simulink model "b6_formation"  (R2021b)
settings: Solver=FixedStepAuto  StartTime=0.0  StopTime=inf  FixedStep=sampleTime  RelTol=1e-3
PreLoadFcn:
  | % Simulation parameters
  | %load exampleMap
  | 
  | % Lidar parameters
  | sensorOffset = [0,0];
  | scanAngles = -pi/2:pi/6:pi/2;
  | maxRange = 0.3;
InitFcn:
  | sampleTime = 0.05;
  | nMedianSize=3;
  | % Robot parameters
  | wheelRadius = 0.0335;
  | robotRadius = 0.116/2;
  | 
  | %角速度坐标
  | ks=1;
  | 
  | % Lidar parameters
  | sensorOffset = [0,0];
  | scanAngles = -pi:pi/36:pi;
  | maxRange = 0.2;
  | 
  | %车初始位置
  | init_pose_1=[1  1.3  pi/2]';
  | init_pose_2=[0.85 1  pi/2]';
  | init_pose_3=[1.15 1  pi/2]';
  | init_pose_4=[0.7  0.7 pi/2]';
  | init_pose_5=[1  0.7 pi/2]';
  | init_pose_6=[1.3 0.7  pi/2]';
  | 
  | %pp算法性能参数
  | Vd_pp=0.2;
  | Wd_pp=pi;
  | dist_pp=0.2;
  | GoalRadius=0.1;
  | numSector=180;
  | rangeDis=[0.1,maxRange];
  | thresholds=[1/360 1/36];
  | safetyDis=0.2;
  | minimumTurningRadius=0.5*robotRadius;
  | recovery_w=0.05;
undefined symbols (not defined in the file): Angular, DiscIntNeverNeededParam, Linear, Pose, Twist
libraries: robotlib x42, dspstat3 x18, mobileRoboticsLib x7, robotmobilelib x6, robotalgslib x6
(part 2 of 5)

== system b6_formation/Subsystem/Car Pose Listener/Subsystem ==
  poseNew : Inport
  poseMsg : Inport  Port=2
  VW_New : Inport  Port=3
  VW_Msg : Inport  Port=4
  DiffSteer Kinematics : Subsystem
      settings: PortSchema="{\"entries\":[{\"content\":{\"sides\":[{\"content\":{\"connectorIds\":[\"In1\",\"In2\"]},\"type\":\"ConnectorPlacement.EquallySpacedRectSide\",\"uuid\":\"0032ed68-1de4-4b1c-b237-9372fedc8a7a\"},{\"content\":{\"connectorIds\":[\"Out1\",\"Out2\",\"Out3\"],\"side\":\"RIGHT\"},\"type\":\"ConnectorPlacement.EquallySpacedRectSide\",\"uuid\":\"d0c861bd-7497-47fe-b183-36da470ee2c6\"},{\"content\":{\"connectorIds\":[\"In3\",\"In4\"],\"side\":\"TOP\"},\"type\":\"ConnectorPlacement.EquallySpacedRectSide\",\"uuid\":\"5b685229-150b-4cb5-b33d-c61d28c4627e\"}]},\"type\":\"ConnectorPlacement.EquallySpacedConnector\",\"uuid\":\"4513c50b-5820-40cb-bb28-cc7c1b1322fe\"}],\"packageUris\":[\"http://schema.mathworks.com/mf0/Connector/R2020b\"],\"version\":\"1.0\"}"
  Median Filter : dspstat3/Median Filter  WindowLength=nMedianSize  SimulateUsing=Interpreted execution
      settings: SourceProductBaseCode=DS
  Median Filter1 : dspstat3/Median Filter  WindowLength=nMedianSize  SimulateUsing=Interpreted execution
      settings: SourceProductBaseCode=DS
  Median Filter2 : dspstat3/Median Filter  WindowLength=nMedianSize  SimulateUsing=Interpreted execution
      settings: SourceProductBaseCode=DS
  Mux7 : Mux  Inputs=3
  Sum : Sum  Inputs=++|
  Sum1 : Sum  Inputs=++|
  sensor2vCar : MATLAB Function  TreatAsAtomicUnit=on
  sensor2vCar4 : MATLAB Function  TreatAsAtomicUnit=on
  pose : Outport
  wires:
  Median Filter2/1 -> Mux7/3
  Median Filter1/1 -> Mux7/2
  Median Filter/1 -> Mux7/1
  sensor2vCar/4(flag) -> DiffSteer Kinematics/3(reset)
  DiffSteer Kinematics/2(y) -> Sum1/2
  sensor2vCar/3(yaw_init) -> DiffSteer Kinematics/4(yaw0)
  sensor2vCar/2(y_init) -> Sum1/1
  sensor2vCar/1(x_init) -> Sum/1
  DiffSteer Kinematics/1(x) -> Sum/2
  VW_New/1 -> sensor2vCar4/1(VW_New)
  Mux7/1 -> pose/1
  Sum/1 -> Median Filter/1
  DiffSteer Kinematics/3(psi) -> Median Filter2/1
  sensor2vCar4/1(V) -> DiffSteer Kinematics/1(u)
  Sum1/1 -> Median Filter1/1
  sensor2vCar4/2(W) -> DiffSteer Kinematics/2(w)
  poseNew/1 -> sensor2vCar/1(poseNew)
  poseMsg/1 -> sensor2vCar/2(poseMsg)
  VW_Msg/1 -> sensor2vCar4/2(VW_Msg)

== system b6_formation/Subsystem/Car Pose Listener1/Subsystem ==
  poseNew : Inport
  poseMsg : Inport  Port=2
  VW_New : Inport  Port=3
  VW_Msg : Inport  Port=4
  DiffSteer Kinematics : Subsystem
      settings: PortSchema="{\"entries\":[{\"content\":{\"sides\":[{\"content\":{\"connectorIds\":[\"In1\",\"In2\"]},\"type\":\"ConnectorPlacement.EquallySpacedRectSide\",\"uuid\":\"0032ed68-1de4-4b1c-b237-9372fedc8a7a\"},{\"content\":{\"connectorIds\":[\"Out1\",\"Out2\",\"Out3\"],\"side\":\"RIGHT\"},\"type\":\"ConnectorPlacement.EquallySpacedRectSide\",\"uuid\":\"d0c861bd-7497-47fe-b183-36da470ee2c6\"},{\"content\":{\"connectorIds\":[\"In3\",\"In4\"],\"side\":\"TOP\"},\"type\":\"ConnectorPlacement.EquallySpacedRectSide\",\"uuid\":\"5b685229-150b-4cb5-b33d-c61d28c4627e\"}]},\"type\":\"ConnectorPlacement.EquallySpacedConnector\",\"uuid\":\"4513c50b-5820-40cb-bb28-cc7c1b1322fe\"}],\"packageUris\":[\"http://schema.mathworks.com/mf0/Connector/R2020b\"],\"version\":\"1.0\"}"
  Median Filter : dspstat3/Median Filter  WindowLength=nMedianSize  SimulateUsing=Interpreted execution
      settings: SourceProductBaseCode=DS
  Median Filter1 : dspstat3/Median Filter  WindowLength=nMedianSize  SimulateUsing=Interpreted execution
      settings: SourceProductBaseCode=DS
  Median Filter2 : dspstat3/Median Filter  WindowLength=nMedianSize  SimulateUsing=Interpreted execution
      settings: SourceProductBaseCode=DS
  Mux7 : Mux  Inputs=3
  Sum : Sum  Inputs=++|
  Sum1 : Sum  Inputs=++|
  sensor2vCar : MATLAB Function  TreatAsAtomicUnit=on
  sensor2vCar4 : MATLAB Function  TreatAsAtomicUnit=on
  pose : Outport
  wires:
  Median Filter2/1 -> Mux7/3
  Median Filter1/1 -> Mux7/2
  Median Filter/1 -> Mux7/1
  sensor2vCar/4(flag) -> DiffSteer Kinematics/3(reset)
  DiffSteer Kinematics/2(y) -> Sum1/2
  sensor2vCar/3(yaw_init) -> DiffSteer Kinematics/4(yaw0)
  sensor2vCar/2(y_init) -> Sum1/1
  sensor2vCar/1(x_init) -> Sum/1
  DiffSteer Kinematics/1(x) -> Sum/2
  VW_New/1 -> sensor2vCar4/1(VW_New)
  Mux7/1 -> pose/1
  Sum/1 -> Median Filter/1
  DiffSteer Kinematics/3(psi) -> Median Filter2/1
  sensor2vCar4/1(V) -> DiffSteer Kinematics/1(u)
  Sum1/1 -> Median Filter1/1
  sensor2vCar4/2(W) -> DiffSteer Kinematics/2(w)
  poseNew/1 -> sensor2vCar/1(poseNew)
  poseMsg/1 -> sensor2vCar/2(poseMsg)
  VW_Msg/1 -> sensor2vCar4/2(VW_Msg)

== system b6_formation/Subsystem/Car Pose Listener2/Subsystem ==
  poseNew : Inport
  poseMsg : Inport  Port=2
  VW_New : Inport  Port=3
  VW_Msg : Inport  Port=4
  DiffSteer Kinematics : Subsystem
      settings: PortSchema="{\"entries\":[{\"content\":{\"sides\":[{\"content\":{\"connectorIds\":[\"In1\",\"In2\"]},\"type\":\"ConnectorPlacement.EquallySpacedRectSide\",\"uuid\":\"0032ed68-1de4-4b1c-b237-9372fedc8a7a\"},{\"content\":{\"connectorIds\":[\"Out1\",\"Out2\",\"Out3\"],\"side\":\"RIGHT\"},\"type\":\"ConnectorPlacement.EquallySpacedRectSide\",\"uuid\":\"d0c861bd-7497-47fe-b183-36da470ee2c6\"},{\"content\":{\"connectorIds\":[\"In3\",\"In4\"],\"side\":\"TOP\"},\"type\":\"ConnectorPlacement.EquallySpacedRectSide\",\"uuid\":\"5b685229-150b-4cb5-b33d-c61d28c4627e\"}]},\"type\":\"ConnectorPlacement.EquallySpacedConnector\",\"uuid\":\"4513c50b-5820-40cb-bb28-cc7c1b1322fe\"}],\"packageUris\":[\"http://schema.mathworks.com/mf0/Connector/R2020b\"],\"version\":\"1.0\"}"
  Median Filter : dspstat3/Median Filter  WindowLength=nMedianSize  SimulateUsing=Interpreted execution
      settings: SourceProductBaseCode=DS
  Median Filter1 : dspstat3/Median Filter  WindowLength=nMedianSize  SimulateUsing=Interpreted execution
      settings: SourceProductBaseCode=DS
  Median Filter2 : dspstat3/Median Filter  WindowLength=nMedianSize  SimulateUsing=Interpreted execution
      settings: SourceProductBaseCode=DS
  Mux7 : Mux  Inputs=3
  Sum : Sum  Inputs=++|
  Sum1 : Sum  Inputs=++|
  sensor2vCar : MATLAB Function  TreatAsAtomicUnit=on
  sensor2vCar4 : MATLAB Function  TreatAsAtomicUnit=on
  pose : Outport
  wires:
  Median Filter2/1 -> Mux7/3
  Median Filter1/1 -> Mux7/2
  Median Filter/1 -> Mux7/1
  sensor2vCar/4(flag) -> DiffSteer Kinematics/3(reset)
  DiffSteer Kinematics/2(y) -> Sum1/2
  sensor2vCar/3(yaw_init) -> DiffSteer Kinematics/4(yaw0)
  sensor2vCar/2(y_init) -> Sum1/1
  sensor2vCar/1(x_init) -> Sum/1
  DiffSteer Kinematics/1(x) -> Sum/2
  VW_New/1 -> sensor2vCar4/1(VW_New)
  Mux7/1 -> pose/1
  Sum/1 -> Median Filter/1
  DiffSteer Kinematics/3(psi) -> Median Filter2/1
  sensor2vCar4/1(V) -> DiffSteer Kinematics/1(u)
  Sum1/1 -> Median Filter1/1
  sensor2vCar4/2(W) -> DiffSteer Kinematics/2(w)
  poseNew/1 -> sensor2vCar/1(poseNew)
  poseMsg/1 -> sensor2vCar/2(poseMsg)
  VW_Msg/1 -> sensor2vCar4/2(VW_Msg)

== system b6_formation/Subsystem/Car Pose Listener3/Subsystem ==
  poseNew : Inport
  poseMsg : Inport  Port=2
  VW_New : Inport  Port=3
  VW_Msg : Inport  Port=4
  DiffSteer Kinematics : Subsystem
      settings: PortSchema="{\"entries\":[{\"content\":{\"sides\":[{\"content\":{\"connectorIds\":[\"In1\",\"In2\"]},\"type\":\"ConnectorPlacement.EquallySpacedRectSide\",\"uuid\":\"0032ed68-1de4-4b1c-b237-9372fedc8a7a\"},{\"content\":{\"connectorIds\":[\"Out1\",\"Out2\",\"Out3\"],\"side\":\"RIGHT\"},\"type\":\"ConnectorPlacement.EquallySpacedRectSide\",\"uuid\":\"d0c861bd-7497-47fe-b183-36da470ee2c6\"},{\"content\":{\"connectorIds\":[\"In3\",\"In4\"],\"side\":\"TOP\"},\"type\":\"ConnectorPlacement.EquallySpacedRectSide\",\"uuid\":\"5b685229-150b-4cb5-b33d-c61d28c4627e\"}]},\"type\":\"ConnectorPlacement.EquallySpacedConnector\",\"uuid\":\"4513c50b-5820-40cb-bb28-cc7c1b1322fe\"}],\"packageUris\":[\"http://schema.mathworks.com/mf0/Connector/R2020b\"],\"version\":\"1.0\"}"
  Median Filter : dspstat3/Median Filter  WindowLength=nMedianSize  SimulateUsing=Interpreted execution
      settings: SourceProductBaseCode=DS
  Median Filter1 : dspstat3/Median Filter  WindowLength=nMedianSize  SimulateUsing=Interpreted execution
      settings: SourceProductBaseCode=DS
  Median Filter2 : dspstat3/Median Filter  WindowLength=nMedianSize  SimulateUsing=Interpreted execution
      settings: SourceProductBaseCode=DS
  Mux7 : Mux  Inputs=3
  Sum : Sum  Inputs=++|
  Sum1 : Sum  Inputs=++|
  sensor2vCar : MATLAB Function  TreatAsAtomicUnit=on
  sensor2vCar4 : MATLAB Function  TreatAsAtomicUnit=on
  pose : Outport
  wires:
  Median Filter2/1 -> Mux7/3
  Median Filter1/1 -> Mux7/2
  Median Filter/1 -> Mux7/1
  sensor2vCar/4(flag) -> DiffSteer Kinematics/3(reset)
  DiffSteer Kinematics/2(y) -> Sum1/2
  sensor2vCar/3(yaw_init) -> DiffSteer Kinematics/4(yaw0)
  sensor2vCar/2(y_init) -> Sum1/1
  sensor2vCar/1(x_init) -> Sum/1
  DiffSteer Kinematics/1(x) -> Sum/2
  VW_New/1 -> sensor2vCar4/1(VW_New)
  Mux7/1 -> pose/1
  Sum/1 -> Median Filter/1
  DiffSteer Kinematics/3(psi) -> Median Filter2/1
  sensor2vCar4/1(V) -> DiffSteer Kinematics/1(u)
  Sum1/1 -> Median Filter1/1
  sensor2vCar4/2(W) -> DiffSteer Kinematics/2(w)
  poseNew/1 -> sensor2vCar/1(poseNew)
  poseMsg/1 -> sensor2vCar/2(poseMsg)
  VW_Msg/1 -> sensor2vCar4/2(VW_Msg)

== system b6_formation/Subsystem/Car Pose Listener4/Subsystem ==
  poseNew : Inport
  poseMsg : Inport  Port=2
  VW_New : Inport  Port=3
  VW_Msg : Inport  Port=4
  DiffSteer Kinematics : Subsystem
      settings: PortSchema="{\"entries\":[{\"content\":{\"sides\":[{\"content\":{\"connectorIds\":[\"In1\",\"In2\"]},\"type\":\"ConnectorPlacement.EquallySpacedRectSide\",\"uuid\":\"0032ed68-1de4-4b1c-b237-9372fedc8a7a\"},{\"content\":{\"connectorIds\":[\"Out1\",\"Out2\",\"Out3\"],\"side\":\"RIGHT\"},\"type\":\"ConnectorPlacement.EquallySpacedRectSide\",\"uuid\":\"d0c861bd-7497-47fe-b183-36da470ee2c6\"},{\"content\":{\"connectorIds\":[\"In3\",\"In4\"],\"side\":\"TOP\"},\"type\":\"ConnectorPlacement.EquallySpacedRectSide\",\"uuid\":\"5b685229-150b-4cb5-b33d-c61d28c4627e\"}]},\"type\":\"ConnectorPlacement.EquallySpacedConnector\",\"uuid\":\"4513c50b-5820-40cb-bb28-cc7c1b1322fe\"}],\"packageUris\":[\"http://schema.mathworks.com/mf0/Connector/R2020b\"],\"version\":\"1.0\"}"
  Median Filter : dspstat3/Median Filter  WindowLength=nMedianSize  SimulateUsing=Interpreted execution
      settings: SourceProductBaseCode=DS
  Median Filter1 : dspstat3/Median Filter  WindowLength=nMedianSize  SimulateUsing=Interpreted execution
      settings: SourceProductBaseCode=DS
  Median Filter2 : dspstat3/Median Filter  WindowLength=nMedianSize  SimulateUsing=Interpreted execution
      settings: SourceProductBaseCode=DS
  Mux7 : Mux  Inputs=3
  Sum : Sum  Inputs=++|
  Sum1 : Sum  Inputs=++|
  sensor2vCar : MATLAB Function  TreatAsAtomicUnit=on
  sensor2vCar4 : MATLAB Function  TreatAsAtomicUnit=on
  pose : Outport
  wires:
  Median Filter2/1 -> Mux7/3
  Median Filter1/1 -> Mux7/2
  Median Filter/1 -> Mux7/1
  sensor2vCar/4(flag) -> DiffSteer Kinematics/3(reset)
  DiffSteer Kinematics/2(y) -> Sum1/2
  sensor2vCar/3(yaw_init) -> DiffSteer Kinematics/4(yaw0)
  sensor2vCar/2(y_init) -> Sum1/1
  sensor2vCar/1(x_init) -> Sum/1
  DiffSteer Kinematics/1(x) -> Sum/2
  VW_New/1 -> sensor2vCar4/1(VW_New)
  Mux7/1 -> pose/1
  Sum/1 -> Median Filter/1
  DiffSteer Kinematics/3(psi) -> Median Filter2/1
  sensor2vCar4/1(V) -> DiffSteer Kinematics/1(u)
  Sum1/1 -> Median Filter1/1
  sensor2vCar4/2(W) -> DiffSteer Kinematics/2(w)
  poseNew/1 -> sensor2vCar/1(poseNew)
  poseMsg/1 -> sensor2vCar/2(poseMsg)
  VW_Msg/1 -> sensor2vCar4/2(VW_Msg)

== system b6_formation/Subsystem/Car Pose Listener5/Subsystem ==
  poseNew : Inport
  poseMsg : Inport  Port=2
  VW_New : Inport  Port=3
  VW_Msg : Inport  Port=4
  DiffSteer Kinematics : Subsystem
      settings: PortSchema="{\"entries\":[{\"content\":{\"sides\":[{\"content\":{\"connectorIds\":[\"In1\",\"In2\"]},\"type\":\"ConnectorPlacement.EquallySpacedRectSide\",\"uuid\":\"0032ed68-1de4-4b1c-b237-9372fedc8a7a\"},{\"content\":{\"connectorIds\":[\"Out1\",\"Out2\",\"Out3\"],\"side\":\"RIGHT\"},\"type\":\"ConnectorPlacement.EquallySpacedRectSide\",\"uuid\":\"d0c861bd-7497-47fe-b183-36da470ee2c6\"},{\"content\":{\"connectorIds\":[\"In3\",\"In4\"],\"side\":\"TOP\"},\"type\":\"ConnectorPlacement.EquallySpacedRectSide\",\"uuid\":\"5b685229-150b-4cb5-b33d-c61d28c4627e\"}]},\"type\":\"ConnectorPlacement.EquallySpacedConnector\",\"uuid\":\"4513c50b-5820-40cb-bb28-cc7c1b1322fe\"}],\"packageUris\":[\"http://schema.mathworks.com/mf0/Connector/R2020b\"],\"version\":\"1.0\"}"
  Median Filter : dspstat3/Median Filter  WindowLength=nMedianSize  SimulateUsing=Interpreted execution
      settings: SourceProductBaseCode=DS
  Median Filter1 : dspstat3/Median Filter  WindowLength=nMedianSize  SimulateUsing=Interpreted execution
      settings: SourceProductBaseCode=DS
  Median Filter2 : dspstat3/Median Filter  WindowLength=nMedianSize  SimulateUsing=Interpreted execution
      settings: SourceProductBaseCode=DS
  Mux7 : Mux  Inputs=3
  Sum : Sum  Inputs=++|
  Sum1 : Sum  Inputs=++|
  sensor2vCar : MATLAB Function  TreatAsAtomicUnit=on
  sensor2vCar4 : MATLAB Function  TreatAsAtomicUnit=on
  pose : Outport
  wires:
  Median Filter2/1 -> Mux7/3
  Median Filter1/1 -> Mux7/2
  Median Filter/1 -> Mux7/1
  sensor2vCar/4(flag) -> DiffSteer Kinematics/3(reset)
  DiffSteer Kinematics/2(y) -> Sum1/2
  sensor2vCar/3(yaw_init) -> DiffSteer Kinematics/4(yaw0)
  sensor2vCar/2(y_init) -> Sum1/1
  sensor2vCar/1(x_init) -> Sum/1
  DiffSteer Kinematics/1(x) -> Sum/2
  VW_New/1 -> sensor2vCar4/1(VW_New)
  Mux7/1 -> pose/1
  Sum/1 -> Median Filter/1
  DiffSteer Kinematics/3(psi) -> Median Filter2/1
  sensor2vCar4/1(V) -> DiffSteer Kinematics/1(u)
  Sum1/1 -> Median Filter1/1
  sensor2vCar4/2(W) -> DiffSteer Kinematics/2(w)
  poseNew/1 -> sensor2vCar/1(poseNew)
  poseMsg/1 -> sensor2vCar/2(poseMsg)
  VW_Msg/1 -> sensor2vCar4/2(VW_Msg)

== system b6_formation/controller/Car1/ppCar ==
  note: Path Following with Obstacle Avoidance in Simulink
  Angels : Inport
  Ranges : Inport  Port=2
  Pose : Inport  Port=3
  WayPoints : Inport  Port=4
  Adjust Velocities to Avoid Obstacles : Subsystem
  Compute Velocity and Heading for Path following : Subsystem
  Constant1 : Constant  Value=scanAngles
  More Info : Subsystem
      settings: OpenFcn=showdemo(bdroot(gcb))
      mask Display: disp('?')
  Outputs : Subsystem
  v : Outport
  w : Outport  Port=2
  wires:
  Outputs/2(w) -> w/1
  Outputs/1(v) -> v/1
  Adjust Velocities to Avoid Obstacles/1(dV) -> Outputs/1(dV)
  WayPoints/1 -> Compute Velocity and Heading for Path following/2(Waypoints)
  Ranges/1 -> Adjust Velocities to Avoid Obstacles/1(Ranges)
  Compute Velocity and Heading for Path following/2(V) -> Outputs/3(V), Adjust Velocities to Avoid Obstacles/4(V)
  Adjust Velocities to Avoid Obstacles/2(dW) -> Outputs/2(dW)
  Pose/1 -> Compute Velocity and Heading for Path following/1(CurrentPose)
  Compute Velocity and Heading for Path following/3(W) -> Outputs/4(W), Adjust Velocities to Avoid Obstacles/5(W)
  Compute Velocity and Heading for Path following/1(TargetDir) -> Adjust Velocities to Avoid Obstacles/3(TargetDir)
  Angels/1 -> Adjust Velocities to Avoid Obstacles/2(Angles)

== system b6_formation/controller/Car2/ppCar ==
  note: Path Following with Obstacle Avoidance in Simulink
  Angels : Inport
  Ranges : Inport  Port=2
  Pose : Inport  Port=3
  WayPoints : Inport  Port=4
  Adjust Velocities to Avoid Obstacles : Subsystem
  Compute Velocity and Heading for Path following : Subsystem
  Constant1 : Constant  Value=scanAngles
  More Info : Subsystem
      settings: OpenFcn=showdemo(bdroot(gcb))
      mask Display: disp('?')
  Outputs : Subsystem
  v : Outport
  w : Outport  Port=2
  wires:
  Angels/1 -> Adjust Velocities to Avoid Obstacles/2(Angles)
  Compute Velocity and Heading for Path following/1(TargetDir) -> Adjust Velocities to Avoid Obstacles/3(TargetDir)
  Compute Velocity and Heading for Path following/3(W) -> Adjust Velocities to Avoid Obstacles/5(W), Outputs/4(W)
  Pose/1 -> Compute Velocity and Heading for Path following/1(CurrentPose)
  Adjust Velocities to Avoid Obstacles/2(dW) -> Outputs/2(dW)
  Compute Velocity and Heading for Path following/2(V) -> Adjust Velocities to Avoid Obstacles/4(V), Outputs/3(V)
  Ranges/1 -> Adjust Velocities to Avoid Obstacles/1(Ranges)
  WayPoints/1 -> Compute Velocity and Heading for Path following/2(Waypoints)
  Adjust Velocities to Avoid Obstacles/1(dV) -> Outputs/1(dV)
  Outputs/1(v) -> v/1
  Outputs/2(w) -> w/1

== system b6_formation/controller/Car3/ppCar ==
  note: Path Following with Obstacle Avoidance in Simulink
  Angels : Inport
  Ranges : Inport  Port=2
  Pose : Inport  Port=3
  WayPoints : Inport  Port=4
  Adjust Velocities to Avoid Obstacles : Subsystem
  Compute Velocity and Heading for Path following : Subsystem
  Constant1 : Constant  Value=scanAngles
  More Info : Subsystem
      settings: OpenFcn=showdemo(bdroot(gcb))
      mask Display: disp('?')
  Outputs : Subsystem
  v : Outport
  w : Outport  Port=2
  wires:
  Outputs/2(w) -> w/1
  Outputs/1(v) -> v/1
  Adjust Velocities to Avoid Obstacles/1(dV) -> Outputs/1(dV)
  WayPoints/1 -> Compute Velocity and Heading for Path following/2(Waypoints)
  Ranges/1 -> Adjust Velocities to Avoid Obstacles/1(Ranges)
  Compute Velocity and Heading for Path following/2(V) -> Outputs/3(V), Adjust Velocities to Avoid Obstacles/4(V)
  Adjust Velocities to Avoid Obstacles/2(dW) -> Outputs/2(dW)
  Pose/1 -> Compute Velocity and Heading for Path following/1(CurrentPose)
  Compute Velocity and Heading for Path following/3(W) -> Outputs/4(W), Adjust Velocities to Avoid Obstacles/5(W)
  Compute Velocity and Heading for Path following/1(TargetDir) -> Adjust Velocities to Avoid Obstacles/3(TargetDir)
  Angels/1 -> Adjust Velocities to Avoid Obstacles/2(Angles)

== system b6_formation/controller/Car4/ppCar ==
  note: Path Following with Obstacle Avoidance in Simulink
  Angels : Inport
  Ranges : Inport  Port=2
  Pose : Inport  Port=3
  WayPoints : Inport  Port=4
  Adjust Velocities to Avoid Obstacles : Subsystem
  Compute Velocity and Heading for Path following : Subsystem
  Constant1 : Constant  Value=scanAngles
  More Info : Subsystem
      settings: OpenFcn=showdemo(bdroot(gcb))
      mask Display: disp('?')
  Outputs : Subsystem
  v : Outport
  w : Outport  Port=2
  wires:
  Angels/1 -> Adjust Velocities to Avoid Obstacles/2(Angles)
  Compute Velocity and Heading for Path following/1(TargetDir) -> Adjust Velocities to Avoid Obstacles/3(TargetDir)
  Compute Velocity and Heading for Path following/3(W) -> Adjust Velocities to Avoid Obstacles/5(W), Outputs/4(W)
  Pose/1 -> Compute Velocity and Heading for Path following/1(CurrentPose)
  Adjust Velocities to Avoid Obstacles/2(dW) -> Outputs/2(dW)
  Compute Velocity and Heading for Path following/2(V) -> Adjust Velocities to Avoid Obstacles/4(V), Outputs/3(V)
  Ranges/1 -> Adjust Velocities to Avoid Obstacles/1(Ranges)
  WayPoints/1 -> Compute Velocity and Heading for Path following/2(Waypoints)
  Adjust Velocities to Avoid Obstacles/1(dV) -> Outputs/1(dV)
  Outputs/1(v) -> v/1
  Outputs/2(w) -> w/1

== system b6_formation/controller/Car5/ppCar ==
  note: Path Following with Obstacle Avoidance in Simulink
  Angels : Inport
  Ranges : Inport  Port=2
  Pose : Inport  Port=3
  WayPoints : Inport  Port=4
  Adjust Velocities to Avoid Obstacles : Subsystem
  Compute Velocity and Heading for Path following : Subsystem
  Constant1 : Constant  Value=scanAngles
  More Info : Subsystem
      settings: OpenFcn=showdemo(bdroot(gcb))
      mask Display: disp('?')
  Outputs : Subsystem
  v : Outport
  w : Outport  Port=2
  wires:
  Outputs/2(w) -> w/1
  Outputs/1(v) -> v/1
  Adjust Velocities to Avoid Obstacles/1(dV) -> Outputs/1(dV)
  WayPoints/1 -> Compute Velocity and Heading for Path following/2(Waypoints)
  Ranges/1 -> Adjust Velocities to Avoid Obstacles/1(Ranges)
  Compute Velocity and Heading for Path following/2(V) -> Outputs/3(V), Adjust Velocities to Avoid Obstacles/4(V)
  Adjust Velocities to Avoid Obstacles/2(dW) -> Outputs/2(dW)
  Pose/1 -> Compute Velocity and Heading for Path following/1(CurrentPose)
  Compute Velocity and Heading for Path following/3(W) -> Outputs/4(W), Adjust Velocities to Avoid Obstacles/5(W)
  Compute Velocity and Heading for Path following/1(TargetDir) -> Adjust Velocities to Avoid Obstacles/3(TargetDir)
  Angels/1 -> Adjust Velocities to Avoid Obstacles/2(Angles)

== system b6_formation/controller/Car6/ppCar ==
  note: Path Following with Obstacle Avoidance in Simulink
  Angels : Inport
  Ranges : Inport  Port=2
  Pose : Inport  Port=3
  WayPoints : Inport  Port=4
  Adjust Velocities to Avoid Obstacles : Subsystem
  Compute Velocity and Heading for Path following : Subsystem
  Constant1 : Constant  Value=scanAngles
  More Info : Subsystem
      settings: OpenFcn=showdemo(bdroot(gcb))
      mask Display: disp('?')
  Outputs : Subsystem
  v : Outport
  w : Outport  Port=2
  wires:
  Angels/1 -> Adjust Velocities to Avoid Obstacles/2(Angles)
  Compute Velocity and Heading for Path following/1(TargetDir) -> Adjust Velocities to Avoid Obstacles/3(TargetDir)
  Compute Velocity and Heading for Path following/3(W) -> Adjust Velocities to Avoid Obstacles/5(W), Outputs/4(W)
  Pose/1 -> Compute Velocity and Heading for Path following/1(CurrentPose)
  Adjust Velocities to Avoid Obstacles/2(dW) -> Outputs/2(dW)
  Compute Velocity and Heading for Path following/2(V) -> Adjust Velocities to Avoid Obstacles/4(V), Outputs/3(V)
  Ranges/1 -> Adjust Velocities to Avoid Obstacles/1(Ranges)
  WayPoints/1 -> Compute Velocity and Heading for Path following/2(Waypoints)
  Adjust Velocities to Avoid Obstacles/1(dV) -> Outputs/1(dV)
  Outputs/1(v) -> v/1
  Outputs/2(w) -> w/1

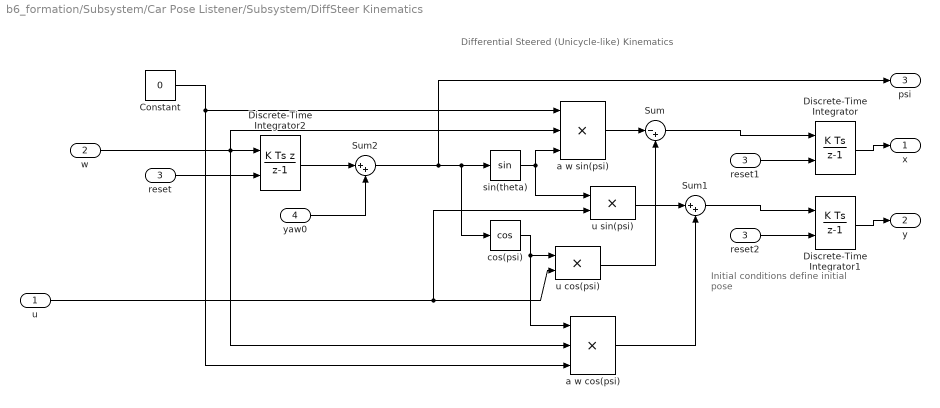
== system b6_formation/Subsystem/Car Pose Listener/Subsystem/DiffSteer Kinematics ==
  note: Initial conditions define
      | initial pose
  note: Differential Steered (Unicycle-like) Kinematics
  u : Inport
  w : Inport  Port=2
  reset : Inport  Port=3
  yaw0 : Inport  Port=4
  Constant : Constant  Value=0
  Discrete-Time Integrator : DiscreteIntegrator  ExternalReset=falling  SampleTime=-1  ICPrevOutput=DiscIntNeverNeededParam  ICPrevScaledInput=DiscIntNeverNeededParam
  Discrete-Time Integrator1 : DiscreteIntegrator  ExternalReset=falling  SampleTime=-1  ICPrevOutput=DiscIntNeverNeededParam  ICPrevScaledInput=DiscIntNeverNeededParam
  Discrete-Time Integrator2 : DiscreteIntegrator  IntegratorMethod=Integration: Backward Euler  ExternalReset=falling  SampleTime=-1  ICPrevOutput=DiscIntNeverNeededParam  ICPrevScaledInput=DiscIntNeverNeededParam
  Sum : Sum  Inputs=|-+  SaturateOnIntegerOverflow=on
  Sum1 : Sum  Inputs=|++  SaturateOnIntegerOverflow=on
  Sum2 : Sum  Inputs=|++
  a w cos(psi) : Product  Inputs=3  SaturateOnIntegerOverflow=on  OutDataTypeStr=Inherit: Same as first input
  a w sin(psi) : Product  Inputs=3  SaturateOnIntegerOverflow=on  OutDataTypeStr=Inherit: Same as first input
  cos(psi) : Trigonometry  Operator=cos
  reset1 : InportShadow  Port=3
  reset2 : InportShadow  Port=3
  sin(theta) : Trigonometry
  u cos(psi) : Product  SaturateOnIntegerOverflow=on  OutDataTypeStr=Inherit: Same as first input
  u sin(psi) : Product  SaturateOnIntegerOverflow=on  OutDataTypeStr=Inherit: Same as first input
  x : Outport
  y : Outport  Port=2
  psi : Outport  Port=3
  wires:
  yaw0/1 -> Sum2/2
  reset2/1 -> Discrete-Time Integrator1/2
  reset1/1 -> Discrete-Time Integrator/2
  reset/1 -> Discrete-Time Integrator2/2
  u sin(psi)/1 -> Sum1/1
  cos(psi)/1 -> u cos(psi)/1, a w cos(psi)/1
  w/1 -> a w cos(psi)/2, a w sin(psi)/2, Discrete-Time Integrator2/1
  Constant/1 -> a w sin(psi)/1, a w cos(psi)/3
  Discrete-Time Integrator/1 -> x/1
  Sum/1 -> Discrete-Time Integrator/1
  sin(theta)/1 -> a w sin(psi)/3, u sin(psi)/1
  a w cos(psi)/1 -> Sum1/2
  Sum2/1 -> psi/1, sin(theta)/1, cos(psi)/1
  u cos(psi)/1 -> Sum/2
  u/1 -> u sin(psi)/2, u cos(psi)/2
  a w sin(psi)/1 -> Sum/1
  Sum1/1 -> Discrete-Time Integrator1/1
  Discrete-Time Integrator1/1 -> y/1
  Discrete-Time Integrator2/1 -> Sum2/1

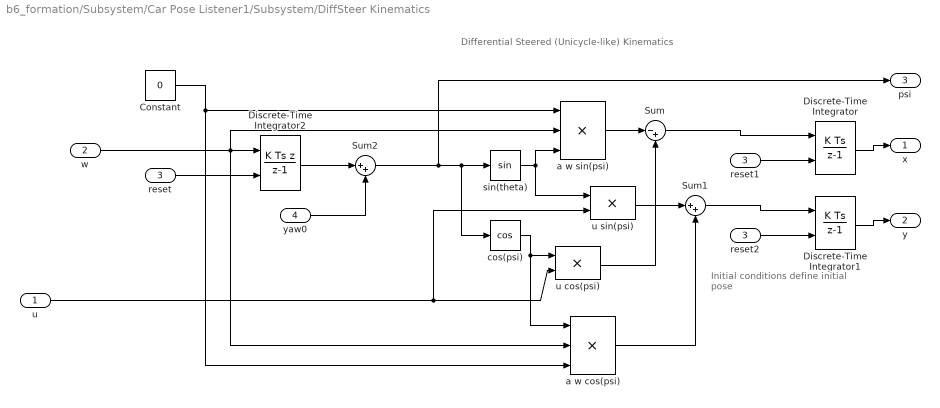
== system b6_formation/Subsystem/Car Pose Listener1/Subsystem/DiffSteer Kinematics ==
  note: Initial conditions define
      | initial pose
  note: Differential Steered (Unicycle-like) Kinematics
  u : Inport
  w : Inport  Port=2
  reset : Inport  Port=3
  yaw0 : Inport  Port=4
  Constant : Constant  Value=0
  Discrete-Time Integrator : DiscreteIntegrator  ExternalReset=falling  SampleTime=-1  ICPrevOutput=DiscIntNeverNeededParam  ICPrevScaledInput=DiscIntNeverNeededParam
  Discrete-Time Integrator1 : DiscreteIntegrator  ExternalReset=falling  SampleTime=-1  ICPrevOutput=DiscIntNeverNeededParam  ICPrevScaledInput=DiscIntNeverNeededParam
  Discrete-Time Integrator2 : DiscreteIntegrator  IntegratorMethod=Integration: Backward Euler  ExternalReset=falling  SampleTime=-1  ICPrevOutput=DiscIntNeverNeededParam  ICPrevScaledInput=DiscIntNeverNeededParam
  Sum : Sum  Inputs=|-+  SaturateOnIntegerOverflow=on
  Sum1 : Sum  Inputs=|++  SaturateOnIntegerOverflow=on
  Sum2 : Sum  Inputs=|++
  a w cos(psi) : Product  Inputs=3  SaturateOnIntegerOverflow=on  OutDataTypeStr=Inherit: Same as first input
  a w sin(psi) : Product  Inputs=3  SaturateOnIntegerOverflow=on  OutDataTypeStr=Inherit: Same as first input
  cos(psi) : Trigonometry  Operator=cos
  reset1 : InportShadow  Port=3
  reset2 : InportShadow  Port=3
  sin(theta) : Trigonometry
  u cos(psi) : Product  SaturateOnIntegerOverflow=on  OutDataTypeStr=Inherit: Same as first input
  u sin(psi) : Product  SaturateOnIntegerOverflow=on  OutDataTypeStr=Inherit: Same as first input
  x : Outport
  y : Outport  Port=2
  psi : Outport  Port=3
  wires:
  yaw0/1 -> Sum2/2
  reset2/1 -> Discrete-Time Integrator1/2
  reset1/1 -> Discrete-Time Integrator/2
  reset/1 -> Discrete-Time Integrator2/2
  u sin(psi)/1 -> Sum1/1
  cos(psi)/1 -> u cos(psi)/1, a w cos(psi)/1
  w/1 -> a w cos(psi)/2, a w sin(psi)/2, Discrete-Time Integrator2/1
  Constant/1 -> a w sin(psi)/1, a w cos(psi)/3
  Discrete-Time Integrator/1 -> x/1
  Sum/1 -> Discrete-Time Integrator/1
  sin(theta)/1 -> a w sin(psi)/3, u sin(psi)/1
  a w cos(psi)/1 -> Sum1/2
  Sum2/1 -> psi/1, sin(theta)/1, cos(psi)/1
  u cos(psi)/1 -> Sum/2
  u/1 -> u sin(psi)/2, u cos(psi)/2
  a w sin(psi)/1 -> Sum/1
  Sum1/1 -> Discrete-Time Integrator1/1
  Discrete-Time Integrator1/1 -> y/1
  Discrete-Time Integrator2/1 -> Sum2/1

== system b6_formation/Subsystem/Car Pose Listener2/Subsystem/DiffSteer Kinematics ==
  note: Initial conditions define
      | initial pose
  note: Differential Steered (Unicycle-like) Kinematics
  u : Inport
  w : Inport  Port=2
  reset : Inport  Port=3
  yaw0 : Inport  Port=4
  Constant : Constant  Value=0
  Discrete-Time Integrator : DiscreteIntegrator  ExternalReset=falling  SampleTime=-1  ICPrevOutput=DiscIntNeverNeededParam  ICPrevScaledInput=DiscIntNeverNeededParam
  Discrete-Time Integrator1 : DiscreteIntegrator  ExternalReset=falling  SampleTime=-1  ICPrevOutput=DiscIntNeverNeededParam  ICPrevScaledInput=DiscIntNeverNeededParam
  Discrete-Time Integrator2 : DiscreteIntegrator  IntegratorMethod=Integration: Backward Euler  ExternalReset=falling  SampleTime=-1  ICPrevOutput=DiscIntNeverNeededParam  ICPrevScaledInput=DiscIntNeverNeededParam
  Sum : Sum  Inputs=|-+  SaturateOnIntegerOverflow=on
  Sum1 : Sum  Inputs=|++  SaturateOnIntegerOverflow=on
  Sum2 : Sum  Inputs=|++
  a w cos(psi) : Product  Inputs=3  SaturateOnIntegerOverflow=on  OutDataTypeStr=Inherit: Same as first input
  a w sin(psi) : Product  Inputs=3  SaturateOnIntegerOverflow=on  OutDataTypeStr=Inherit: Same as first input
  cos(psi) : Trigonometry  Operator=cos
  reset1 : InportShadow  Port=3
  reset2 : InportShadow  Port=3
  sin(theta) : Trigonometry
  u cos(psi) : Product  SaturateOnIntegerOverflow=on  OutDataTypeStr=Inherit: Same as first input
  u sin(psi) : Product  SaturateOnIntegerOverflow=on  OutDataTypeStr=Inherit: Same as first input
  x : Outport
  y : Outport  Port=2
  psi : Outport  Port=3
  wires:
  yaw0/1 -> Sum2/2
  reset2/1 -> Discrete-Time Integrator1/2
  reset1/1 -> Discrete-Time Integrator/2
  reset/1 -> Discrete-Time Integrator2/2
  u sin(psi)/1 -> Sum1/1
  cos(psi)/1 -> u cos(psi)/1, a w cos(psi)/1
  w/1 -> a w cos(psi)/2, a w sin(psi)/2, Discrete-Time Integrator2/1
  Constant/1 -> a w sin(psi)/1, a w cos(psi)/3
  Discrete-Time Integrator/1 -> x/1
  Sum/1 -> Discrete-Time Integrator/1
  sin(theta)/1 -> a w sin(psi)/3, u sin(psi)/1
  a w cos(psi)/1 -> Sum1/2
  Sum2/1 -> psi/1, sin(theta)/1, cos(psi)/1
  u cos(psi)/1 -> Sum/2
  u/1 -> u sin(psi)/2, u cos(psi)/2
  a w sin(psi)/1 -> Sum/1
  Sum1/1 -> Discrete-Time Integrator1/1
  Discrete-Time Integrator1/1 -> y/1
  Discrete-Time Integrator2/1 -> Sum2/1

== system b6_formation/Subsystem/Car Pose Listener3/Subsystem/DiffSteer Kinematics ==
  note: Initial conditions define
      | initial pose
  note: Differential Steered (Unicycle-like) Kinematics
  u : Inport
  w : Inport  Port=2
  reset : Inport  Port=3
  yaw0 : Inport  Port=4
  Constant : Constant  Value=0
  Discrete-Time Integrator : DiscreteIntegrator  ExternalReset=falling  SampleTime=-1  ICPrevOutput=DiscIntNeverNeededParam  ICPrevScaledInput=DiscIntNeverNeededParam
  Discrete-Time Integrator1 : DiscreteIntegrator  ExternalReset=falling  SampleTime=-1  ICPrevOutput=DiscIntNeverNeededParam  ICPrevScaledInput=DiscIntNeverNeededParam
  Discrete-Time Integrator2 : DiscreteIntegrator  IntegratorMethod=Integration: Backward Euler  ExternalReset=falling  SampleTime=-1  ICPrevOutput=DiscIntNeverNeededParam  ICPrevScaledInput=DiscIntNeverNeededParam
  Sum : Sum  Inputs=|-+  SaturateOnIntegerOverflow=on
  Sum1 : Sum  Inputs=|++  SaturateOnIntegerOverflow=on
  Sum2 : Sum  Inputs=|++
  a w cos(psi) : Product  Inputs=3  SaturateOnIntegerOverflow=on  OutDataTypeStr=Inherit: Same as first input
  a w sin(psi) : Product  Inputs=3  SaturateOnIntegerOverflow=on  OutDataTypeStr=Inherit: Same as first input
  cos(psi) : Trigonometry  Operator=cos
  reset1 : InportShadow  Port=3
  reset2 : InportShadow  Port=3
  sin(theta) : Trigonometry
  u cos(psi) : Product  SaturateOnIntegerOverflow=on  OutDataTypeStr=Inherit: Same as first input
  u sin(psi) : Product  SaturateOnIntegerOverflow=on  OutDataTypeStr=Inherit: Same as first input
  x : Outport
  y : Outport  Port=2
  psi : Outport  Port=3
  wires:
  yaw0/1 -> Sum2/2
  reset2/1 -> Discrete-Time Integrator1/2
  reset1/1 -> Discrete-Time Integrator/2
  reset/1 -> Discrete-Time Integrator2/2
  u sin(psi)/1 -> Sum1/1
  cos(psi)/1 -> u cos(psi)/1, a w cos(psi)/1
  w/1 -> a w cos(psi)/2, a w sin(psi)/2, Discrete-Time Integrator2/1
  Constant/1 -> a w sin(psi)/1, a w cos(psi)/3
  Discrete-Time Integrator/1 -> x/1
  Sum/1 -> Discrete-Time Integrator/1
  sin(theta)/1 -> a w sin(psi)/3, u sin(psi)/1
  a w cos(psi)/1 -> Sum1/2
  Sum2/1 -> psi/1, sin(theta)/1, cos(psi)/1
  u cos(psi)/1 -> Sum/2
  u/1 -> u sin(psi)/2, u cos(psi)/2
  a w sin(psi)/1 -> Sum/1
  Sum1/1 -> Discrete-Time Integrator1/1
  Discrete-Time Integrator1/1 -> y/1
  Discrete-Time Integrator2/1 -> Sum2/1

== system b6_formation/Subsystem/Car Pose Listener4/Subsystem/DiffSteer Kinematics ==
  note: Initial conditions define
      | initial pose
  note: Differential Steered (Unicycle-like) Kinematics
  u : Inport
  w : Inport  Port=2
  reset : Inport  Port=3
  yaw0 : Inport  Port=4
  Constant : Constant  Value=0
  Discrete-Time Integrator : DiscreteIntegrator  ExternalReset=falling  SampleTime=-1  ICPrevOutput=DiscIntNeverNeededParam  ICPrevScaledInput=DiscIntNeverNeededParam
  Discrete-Time Integrator1 : DiscreteIntegrator  ExternalReset=falling  SampleTime=-1  ICPrevOutput=DiscIntNeverNeededParam  ICPrevScaledInput=DiscIntNeverNeededParam
  Discrete-Time Integrator2 : DiscreteIntegrator  IntegratorMethod=Integration: Backward Euler  ExternalReset=falling  SampleTime=-1  ICPrevOutput=DiscIntNeverNeededParam  ICPrevScaledInput=DiscIntNeverNeededParam
  Sum : Sum  Inputs=|-+  SaturateOnIntegerOverflow=on
  Sum1 : Sum  Inputs=|++  SaturateOnIntegerOverflow=on
  Sum2 : Sum  Inputs=|++
  a w cos(psi) : Product  Inputs=3  SaturateOnIntegerOverflow=on  OutDataTypeStr=Inherit: Same as first input
  a w sin(psi) : Product  Inputs=3  SaturateOnIntegerOverflow=on  OutDataTypeStr=Inherit: Same as first input
  cos(psi) : Trigonometry  Operator=cos
  reset1 : InportShadow  Port=3
  reset2 : InportShadow  Port=3
  sin(theta) : Trigonometry
  u cos(psi) : Product  SaturateOnIntegerOverflow=on  OutDataTypeStr=Inherit: Same as first input
  u sin(psi) : Product  SaturateOnIntegerOverflow=on  OutDataTypeStr=Inherit: Same as first input
  x : Outport
  y : Outport  Port=2
  psi : Outport  Port=3
  wires:
  yaw0/1 -> Sum2/2
  reset2/1 -> Discrete-Time Integrator1/2
  reset1/1 -> Discrete-Time Integrator/2
  reset/1 -> Discrete-Time Integrator2/2
  u sin(psi)/1 -> Sum1/1
  cos(psi)/1 -> u cos(psi)/1, a w cos(psi)/1
  w/1 -> a w cos(psi)/2, a w sin(psi)/2, Discrete-Time Integrator2/1
  Constant/1 -> a w sin(psi)/1, a w cos(psi)/3
  Discrete-Time Integrator/1 -> x/1
  Sum/1 -> Discrete-Time Integrator/1
  sin(theta)/1 -> a w sin(psi)/3, u sin(psi)/1
  a w cos(psi)/1 -> Sum1/2
  Sum2/1 -> psi/1, sin(theta)/1, cos(psi)/1
  u cos(psi)/1 -> Sum/2
  u/1 -> u sin(psi)/2, u cos(psi)/2
  a w sin(psi)/1 -> Sum/1
  Sum1/1 -> Discrete-Time Integrator1/1
  Discrete-Time Integrator1/1 -> y/1
  Discrete-Time Integrator2/1 -> Sum2/1

== system b6_formation/Subsystem/Car Pose Listener5/Subsystem/DiffSteer Kinematics ==
  note: Initial conditions define
      | initial pose
  note: Differential Steered (Unicycle-like) Kinematics
  u : Inport
  w : Inport  Port=2
  reset : Inport  Port=3
  yaw0 : Inport  Port=4
  Constant : Constant  Value=0
  Discrete-Time Integrator : DiscreteIntegrator  ExternalReset=falling  SampleTime=-1  ICPrevOutput=DiscIntNeverNeededParam  ICPrevScaledInput=DiscIntNeverNeededParam
  Discrete-Time Integrator1 : DiscreteIntegrator  ExternalReset=falling  SampleTime=-1  ICPrevOutput=DiscIntNeverNeededParam  ICPrevScaledInput=DiscIntNeverNeededParam
  Discrete-Time Integrator2 : DiscreteIntegrator  IntegratorMethod=Integration: Backward Euler  ExternalReset=falling  SampleTime=-1  ICPrevOutput=DiscIntNeverNeededParam  ICPrevScaledInput=DiscIntNeverNeededParam
  Sum : Sum  Inputs=|-+  SaturateOnIntegerOverflow=on
  Sum1 : Sum  Inputs=|++  SaturateOnIntegerOverflow=on
  Sum2 : Sum  Inputs=|++
  a w cos(psi) : Product  Inputs=3  SaturateOnIntegerOverflow=on  OutDataTypeStr=Inherit: Same as first input
  a w sin(psi) : Product  Inputs=3  SaturateOnIntegerOverflow=on  OutDataTypeStr=Inherit: Same as first input
  cos(psi) : Trigonometry  Operator=cos
  reset1 : InportShadow  Port=3
  reset2 : InportShadow  Port=3
  sin(theta) : Trigonometry
  u cos(psi) : Product  SaturateOnIntegerOverflow=on  OutDataTypeStr=Inherit: Same as first input
  u sin(psi) : Product  SaturateOnIntegerOverflow=on  OutDataTypeStr=Inherit: Same as first input
  x : Outport
  y : Outport  Port=2
  psi : Outport  Port=3
  wires:
  yaw0/1 -> Sum2/2
  reset2/1 -> Discrete-Time Integrator1/2
  reset1/1 -> Discrete-Time Integrator/2
  reset/1 -> Discrete-Time Integrator2/2
  u sin(psi)/1 -> Sum1/1
  cos(psi)/1 -> u cos(psi)/1, a w cos(psi)/1
  w/1 -> a w cos(psi)/2, a w sin(psi)/2, Discrete-Time Integrator2/1
  Constant/1 -> a w sin(psi)/1, a w cos(psi)/3
  Discrete-Time Integrator/1 -> x/1
  Sum/1 -> Discrete-Time Integrator/1
  sin(theta)/1 -> a w sin(psi)/3, u sin(psi)/1
  a w cos(psi)/1 -> Sum1/2
  Sum2/1 -> psi/1, sin(theta)/1, cos(psi)/1
  u cos(psi)/1 -> Sum/2
  u/1 -> u sin(psi)/2, u cos(psi)/2
  a w sin(psi)/1 -> Sum/1
  Sum1/1 -> Discrete-Time Integrator1/1
  Discrete-Time Integrator1/1 -> y/1
  Discrete-Time Integrator2/1 -> Sum2/1

== system b6_formation/controller/Car1/ppCar/Adjust Velocities to Avoid Obstacles ==
  note: Based on proposed steering direction, evaluate feasible velocities (linear and angular).
      | 				Switch to recovery behavior if no feasible steering direction.
  Ranges : Inport
  Angles : Inport  Port=2
  TargetDir : Inport  Port=3
  V : Inport  Port=4
  W : Inport  Port=5
  If : If  IfExpression=u1 == 1
  Merge : Merge
  Merge1 : Merge
  Path Following : Subsystem  TreatAsAtomicUnit=on
  Recovery : Subsystem  TreatAsAtomicUnit=on
  Relational Operator : RelationalOperator  Operator=isNaN  OutDataTypeStr=boolean  RndMeth=Simplest
  Vector Field Histogram : robotalgslib/Vector Field Histogram  NumAngularSectors=numSector  DistanceLimits=rangeDis  HistogramThresholds=thresholds  RobotRadius=vehicleRadius  SafetyDistance=safetyDis  MinTurningRadius=minimumTurningRadius  SimulateUsing=Code generation  TargetDirectionWeight=50  CurrentDirectionWeight=20  PreviousDirectionWeight=20
      settings: SourceProductBaseCode=NV,RO
  dV : Outport  VectorParamsAs1DForOutWhenUnconnected=off
  dW : Outport  Port=2  VectorParamsAs1DForOutWhenUnconnected=off
  wires:
  Path Following/1(dV) -> Merge/2
  Recovery/1(dV) -> Merge/1
  Path Following/2(dW) -> Merge1/2
  Recovery/2(dW) -> Merge1/1
  If/2 -> Path Following/Action
  If/1 -> Recovery/Action
  Ranges/1 -> Vector Field Histogram/1
  TargetDir/1 -> Vector Field Histogram/3
  Merge/1 -> dV/1
  Angles/1 -> Vector Field Histogram/2
  Relational Operator/1 -> If/1
  W/1 -> Path Following/3(AngularVelocity), Recovery/2(AngularVelocity)
  Vector Field Histogram/1 -> Path Following/1(SteeringDirection), Relational Operator/1
  V/1 -> Path Following/2(V), Recovery/1(LinearVelocity)
  Merge1/1 -> dW/1

== system b6_formation/controller/Car1/ppCar/Compute Velocity and Heading for Path following ==
  CurrentPose : Inport
  Waypoints : Inport  Port=2
  Car1 : Subsystem
  TargetDir : Outport  VectorParamsAs1DForOutWhenUnconnected=off
  V : Outport  Port=2  VectorParamsAs1DForOutWhenUnconnected=off
  W : Outport  Port=3  VectorParamsAs1DForOutWhenUnconnected=off
  wires:
  Car1/3(targetdir) -> TargetDir/1
  Car1/2(W) -> W/1
  Car1/1(V) -> V/1
  Waypoints/1 -> Car1/2(waypoint)
  CurrentPose/1 -> Car1/1(pose)

== system b6_formation/controller/Car1/ppCar/More Info ==

== system b6_formation/controller/Car1/ppCar/Outputs ==
  dV : Inport
  dW : Inport  Port=2
  V : Inport  Port=3
  W : Inport  Port=4
  Add : Sum
  Add1 : Sum
  v : Outport
  w : Outport  Port=2
  wires:
  Add/1 -> v/1
  Add1/1 -> w/1
  dW/1 -> Add1/1
  dV/1 -> Add/1
  W/1 -> Add1/2
  V/1 -> Add/2

== system b6_formation/controller/Car2/ppCar/Adjust Velocities to Avoid Obstacles ==
  note: Based on proposed steering direction, evaluate feasible velocities (linear and angular).
      | 				Switch to recovery behavior if no feasible steering direction.
  Ranges : Inport
  Angles : Inport  Port=2
  TargetDir : Inport  Port=3
  V : Inport  Port=4
  W : Inport  Port=5
  If : If  IfExpression=u1 == 1
  Merge : Merge
  Merge1 : Merge
  Path Following : Subsystem  TreatAsAtomicUnit=on
  Recovery : Subsystem  TreatAsAtomicUnit=on
  Relational Operator : RelationalOperator  Operator=isNaN  OutDataTypeStr=boolean  RndMeth=Simplest
  Vector Field Histogram : robotalgslib/Vector Field Histogram  NumAngularSectors=numSector  DistanceLimits=rangeDis  HistogramThresholds=thresholds  RobotRadius=vehicleRadius  SafetyDistance=safetyDis  MinTurningRadius=minimumTurningRadius  SimulateUsing=Code generation  TargetDirectionWeight=50  CurrentDirectionWeight=20  PreviousDirectionWeight=20
      settings: SourceProductBaseCode=NV,RO
  dV : Outport  VectorParamsAs1DForOutWhenUnconnected=off
  dW : Outport  Port=2  VectorParamsAs1DForOutWhenUnconnected=off
  wires:
  Merge1/1 -> dW/1
  V/1 -> Recovery/1(LinearVelocity), Path Following/2(V)
  Vector Field Histogram/1 -> Relational Operator/1, Path Following/1(SteeringDirection)
  W/1 -> Recovery/2(AngularVelocity), Path Following/3(AngularVelocity)
  Relational Operator/1 -> If/1
  Angles/1 -> Vector Field Histogram/2
  Merge/1 -> dV/1
  TargetDir/1 -> Vector Field Histogram/3
  Ranges/1 -> Vector Field Histogram/1
  If/1 -> Recovery/Action
  If/2 -> Path Following/Action
  Recovery/2(dW) -> Merge1/1
  Path Following/2(dW) -> Merge1/2
  Recovery/1(dV) -> Merge/1
  Path Following/1(dV) -> Merge/2

== system b6_formation/controller/Car2/ppCar/Compute Velocity and Heading for Path following ==
  CurrentPose : Inport
  Waypoints : Inport  Port=2
  Car1 : Subsystem
  TargetDir : Outport  VectorParamsAs1DForOutWhenUnconnected=off
  V : Outport  Port=2  VectorParamsAs1DForOutWhenUnconnected=off
  W : Outport  Port=3  VectorParamsAs1DForOutWhenUnconnected=off
  wires:
  CurrentPose/1 -> Car1/1(pose)
  Waypoints/1 -> Car1/2(waypoint)
  Car1/1(V) -> V/1
  Car1/2(W) -> W/1
  Car1/3(targetdir) -> TargetDir/1

== system b6_formation/controller/Car2/ppCar/More Info ==

== system b6_formation/controller/Car2/ppCar/Outputs ==
  dV : Inport
  dW : Inport  Port=2
  V : Inport  Port=3
  W : Inport  Port=4
  Add : Sum
  Add1 : Sum
  v : Outport
  w : Outport  Port=2
  wires:
  V/1 -> Add/2
  W/1 -> Add1/2
  dV/1 -> Add/1
  dW/1 -> Add1/1
  Add1/1 -> w/1
  Add/1 -> v/1

== system b6_formation/controller/Car3/ppCar/Adjust Velocities to Avoid Obstacles ==
  note: Based on proposed steering direction, evaluate feasible velocities (linear and angular).
      | 				Switch to recovery behavior if no feasible steering direction.
  Ranges : Inport
  Angles : Inport  Port=2
  TargetDir : Inport  Port=3
  V : Inport  Port=4
  W : Inport  Port=5
  If : If  IfExpression=u1 == 1
  Merge : Merge
  Merge1 : Merge
  Path Following : Subsystem  TreatAsAtomicUnit=on
  Recovery : Subsystem  TreatAsAtomicUnit=on
  Relational Operator : RelationalOperator  Operator=isNaN  OutDataTypeStr=boolean  RndMeth=Simplest
  Vector Field Histogram : robotalgslib/Vector Field Histogram  NumAngularSectors=numSector  DistanceLimits=rangeDis  HistogramThresholds=thresholds  RobotRadius=vehicleRadius  SafetyDistance=safetyDis  MinTurningRadius=minimumTurningRadius  SimulateUsing=Code generation  TargetDirectionWeight=50  CurrentDirectionWeight=20  PreviousDirectionWeight=20
      settings: SourceProductBaseCode=NV,RO
  dV : Outport  VectorParamsAs1DForOutWhenUnconnected=off
  dW : Outport  Port=2  VectorParamsAs1DForOutWhenUnconnected=off
  wires:
  Path Following/1(dV) -> Merge/2
  Recovery/1(dV) -> Merge/1
  Path Following/2(dW) -> Merge1/2
  Recovery/2(dW) -> Merge1/1
  If/2 -> Path Following/Action
  If/1 -> Recovery/Action
  Ranges/1 -> Vector Field Histogram/1
  TargetDir/1 -> Vector Field Histogram/3
  Merge/1 -> dV/1
  Angles/1 -> Vector Field Histogram/2
  Relational Operator/1 -> If/1
  W/1 -> Path Following/3(AngularVelocity), Recovery/2(AngularVelocity)
  Vector Field Histogram/1 -> Path Following/1(SteeringDirection), Relational Operator/1
  V/1 -> Path Following/2(V), Recovery/1(LinearVelocity)
  Merge1/1 -> dW/1

== system b6_formation/controller/Car3/ppCar/Compute Velocity and Heading for Path following ==
  CurrentPose : Inport
  Waypoints : Inport  Port=2
  Car1 : Subsystem
  TargetDir : Outport  VectorParamsAs1DForOutWhenUnconnected=off
  V : Outport  Port=2  VectorParamsAs1DForOutWhenUnconnected=off
  W : Outport  Port=3  VectorParamsAs1DForOutWhenUnconnected=off
  wires:
  Car1/3(targetdir) -> TargetDir/1
  Car1/2(W) -> W/1
  Car1/1(V) -> V/1
  Waypoints/1 -> Car1/2(waypoint)
  CurrentPose/1 -> Car1/1(pose)

== system b6_formation/controller/Car3/ppCar/More Info ==

== system b6_formation/controller/Car3/ppCar/Outputs ==
  dV : Inport
  dW : Inport  Port=2
  V : Inport  Port=3
  W : Inport  Port=4
  Add : Sum
  Add1 : Sum
  v : Outport
  w : Outport  Port=2
  wires:
  Add/1 -> v/1
  Add1/1 -> w/1
  dW/1 -> Add1/1
  dV/1 -> Add/1
  W/1 -> Add1/2
  V/1 -> Add/2

== system b6_formation/controller/Car4/ppCar/Adjust Velocities to Avoid Obstacles ==
  note: Based on proposed steering direction, evaluate feasible velocities (linear and angular).
      | 				Switch to recovery behavior if no feasible steering direction.
  Ranges : Inport
  Angles : Inport  Port=2
  TargetDir : Inport  Port=3
  V : Inport  Port=4
  W : Inport  Port=5
  If : If  IfExpression=u1 == 1
  Merge : Merge
  Merge1 : Merge
  Path Following : Subsystem  TreatAsAtomicUnit=on
  Recovery : Subsystem  TreatAsAtomicUnit=on
  Relational Operator : RelationalOperator  Operator=isNaN  OutDataTypeStr=boolean  RndMeth=Simplest
  Vector Field Histogram : robotalgslib/Vector Field Histogram  NumAngularSectors=numSector  DistanceLimits=rangeDis  HistogramThresholds=thresholds  RobotRadius=vehicleRadius  SafetyDistance=safetyDis  MinTurningRadius=minimumTurningRadius  SimulateUsing=Code generation  TargetDirectionWeight=50  CurrentDirectionWeight=20  PreviousDirectionWeight=20
      settings: SourceProductBaseCode=NV,RO
  dV : Outport  VectorParamsAs1DForOutWhenUnconnected=off
  dW : Outport  Port=2  VectorParamsAs1DForOutWhenUnconnected=off
  wires:
  Merge1/1 -> dW/1
  V/1 -> Recovery/1(LinearVelocity), Path Following/2(V)
  Vector Field Histogram/1 -> Relational Operator/1, Path Following/1(SteeringDirection)
  W/1 -> Recovery/2(AngularVelocity), Path Following/3(AngularVelocity)
  Relational Operator/1 -> If/1
  Angles/1 -> Vector Field Histogram/2
  Merge/1 -> dV/1
  TargetDir/1 -> Vector Field Histogram/3
  Ranges/1 -> Vector Field Histogram/1
  If/1 -> Recovery/Action
  If/2 -> Path Following/Action
  Recovery/2(dW) -> Merge1/1
  Path Following/2(dW) -> Merge1/2
  Recovery/1(dV) -> Merge/1
  Path Following/1(dV) -> Merge/2

== system b6_formation/controller/Car4/ppCar/Compute Velocity and Heading for Path following ==
  CurrentPose : Inport
  Waypoints : Inport  Port=2
  Car1 : Subsystem
  TargetDir : Outport  VectorParamsAs1DForOutWhenUnconnected=off
  V : Outport  Port=2  VectorParamsAs1DForOutWhenUnconnected=off
  W : Outport  Port=3  VectorParamsAs1DForOutWhenUnconnected=off
  wires:
  CurrentPose/1 -> Car1/1(pose)
  Waypoints/1 -> Car1/2(waypoint)
  Car1/1(V) -> V/1
  Car1/2(W) -> W/1
  Car1/3(targetdir) -> TargetDir/1

== system b6_formation/controller/Car4/ppCar/More Info ==

== system b6_formation/controller/Car4/ppCar/Outputs ==
  dV : Inport
  dW : Inport  Port=2
  V : Inport  Port=3
  W : Inport  Port=4
  Add : Sum
  Add1 : Sum
  v : Outport
  w : Outport  Port=2
  wires:
  V/1 -> Add/2
  W/1 -> Add1/2
  dV/1 -> Add/1
  dW/1 -> Add1/1
  Add1/1 -> w/1
  Add/1 -> v/1

== system b6_formation/controller/Car5/ppCar/Adjust Velocities to Avoid Obstacles ==
  note: Based on proposed steering direction, evaluate feasible velocities (linear and angular).
      | 				Switch to recovery behavior if no feasible steering direction.
  Ranges : Inport
  Angles : Inport  Port=2
  TargetDir : Inport  Port=3
  V : Inport  Port=4
  W : Inport  Port=5
  If : If  IfExpression=u1 == 1
  Merge : Merge
  Merge1 : Merge
  Path Following : Subsystem  TreatAsAtomicUnit=on
  Recovery : Subsystem  TreatAsAtomicUnit=on
  Relational Operator : RelationalOperator  Operator=isNaN  OutDataTypeStr=boolean  RndMeth=Simplest
  Vector Field Histogram : robotalgslib/Vector Field Histogram  NumAngularSectors=numSector  DistanceLimits=rangeDis  HistogramThresholds=thresholds  RobotRadius=vehicleRadius  SafetyDistance=safetyDis  MinTurningRadius=minimumTurningRadius  SimulateUsing=Code generation  TargetDirectionWeight=50  CurrentDirectionWeight=20  PreviousDirectionWeight=20
      settings: SourceProductBaseCode=NV,RO
  dV : Outport  VectorParamsAs1DForOutWhenUnconnected=off
  dW : Outport  Port=2  VectorParamsAs1DForOutWhenUnconnected=off
  wires:
  Path Following/1(dV) -> Merge/2
  Recovery/1(dV) -> Merge/1
  Path Following/2(dW) -> Merge1/2
  Recovery/2(dW) -> Merge1/1
  If/2 -> Path Following/Action
  If/1 -> Recovery/Action
  Ranges/1 -> Vector Field Histogram/1
  TargetDir/1 -> Vector Field Histogram/3
  Merge/1 -> dV/1
  Angles/1 -> Vector Field Histogram/2
  Relational Operator/1 -> If/1
  W/1 -> Path Following/3(AngularVelocity), Recovery/2(AngularVelocity)
  Vector Field Histogram/1 -> Path Following/1(SteeringDirection), Relational Operator/1
  V/1 -> Path Following/2(V), Recovery/1(LinearVelocity)
  Merge1/1 -> dW/1

== system b6_formation/controller/Car5/ppCar/Compute Velocity and Heading for Path following ==
  CurrentPose : Inport
  Waypoints : Inport  Port=2
  Car1 : Subsystem
  TargetDir : Outport  VectorParamsAs1DForOutWhenUnconnected=off
  V : Outport  Port=2  VectorParamsAs1DForOutWhenUnconnected=off
  W : Outport  Port=3  VectorParamsAs1DForOutWhenUnconnected=off
  wires:
  Car1/3(targetdir) -> TargetDir/1
  Car1/2(W) -> W/1
  Car1/1(V) -> V/1
  Waypoints/1 -> Car1/2(waypoint)
  CurrentPose/1 -> Car1/1(pose)

== system b6_formation/controller/Car5/ppCar/More Info ==
